simulink model "scheme1_1"  (R2021a)
settings: Solver=VariableStepAuto  StartTime=0.0  StopTime=10.0  RelTol=1e-3
values from neighbouring files (symbols this model uses):
  k = 6    [exercise1.m]
  T_1 = 5.9    [exercise1.m]
  T_2 = 0.8    [exercise1.m]
  Tp = 0.01    [exercise1.m]
settings Model: Creator=AgraWoodAdmin  LastModifiedBy=AgraWoodAdmin

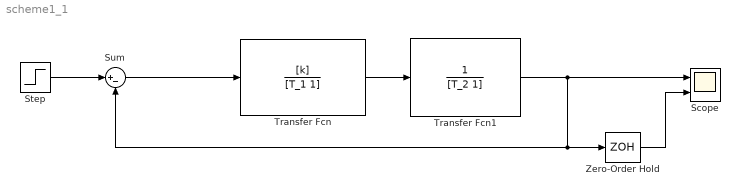
== system scheme1_1 ==
  Scope : Scope  NumInputPorts=2
  Step : Step  Time=0  SampleTime=0
  Sum : Sum  Inputs=|+-
  Transfer Fcn : TransferFcn  Numerator=[k]  Denominator=[T_1 1]
  Transfer Fcn1 : TransferFcn  Denominator=[T_2 1]
  Zero-Order Hold : ZeroOrderHold  SampleTime=Tp
  wires:
  Zero-Order Hold/1 -> Scope/2
  Step/1 -> Sum/1
  Sum/1 -> Transfer Fcn/1
  Transfer Fcn1/1 -> Zero-Order Hold/1, Sum/2, Scope/1
  Transfer Fcn/1 -> Transfer Fcn1/1
